simulink model "EGRVlv_DD"  (R2020b)
settings: configuration reference "cs_ert" (kept outside this file)
values from neighbouring files (symbols this model uses):
  EGRVlv_rPwmOutMax_C = 0.0    [EGRVlv_DD.sldd]
  EGRVlv_rPwmOutMin_C = 0.0    [EGRVlv_DD.sldd]
  EGRVlv_tiPs_C = 0.0    [EGRVlv_DD.sldd]
libraries: simulink x1
settings Model: DataDictionary=EGRVlv_DD.sldd  EnableAccessToBaseWorkspace=off  Creator=zhoutinglin  LastModifiedBy=zhoutinglin
settings ConfigSetRef: SourceName=cs_ert

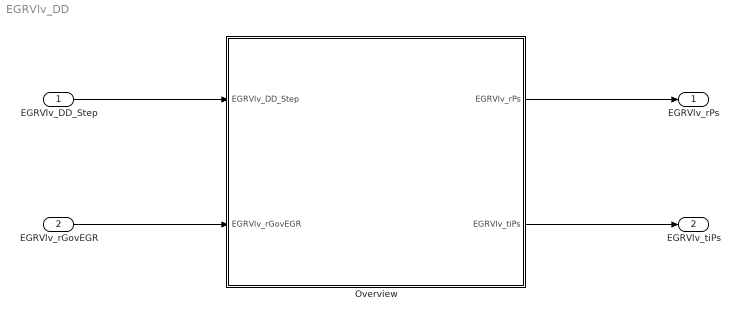
== system EGRVlv_DD ==
  EGRVlv_DD_Step : Inport  OutputFunctionCall=on
  EGRVlv_rGovEGR : Inport  Description=Control value for the EGR valve  Port=2  OutMin=-100  OutMax=100  OutDataTypeStr=DutyCycle  Unit=%  PortDimensions=[1 1]
  Overview : Subsystem
  EGRVlv_rPs : Outport  Description=Duty cycle to power stage  OutMin=-100  OutMax=100  OutDataTypeStr=DutyCycle  Unit=%  PortDimensions=[1 1]  VectorParamsAs1DForOutWhenUnconnected=off
  EGRVlv_tiPs : Outport  Description=signal period duration  Port=2  OutMin=0  OutMax=1000  OutDataTypeStr=Period_us1  Unit=us  PortDimensions=[1 1]  VectorParamsAs1DForOutWhenUnconnected=off
  wires:
  EGRVlv_DD_Step/1 -> Overview/1(EGRVlv_DD_Step)
  EGRVlv_rGovEGR/1 -> Overview/2(EGRVlv_rGovEGR)
  Overview/1(EGRVlv_rPs) -> EGRVlv_rPs/1
  Overview/2(EGRVlv_tiPs) -> EGRVlv_tiPs/1

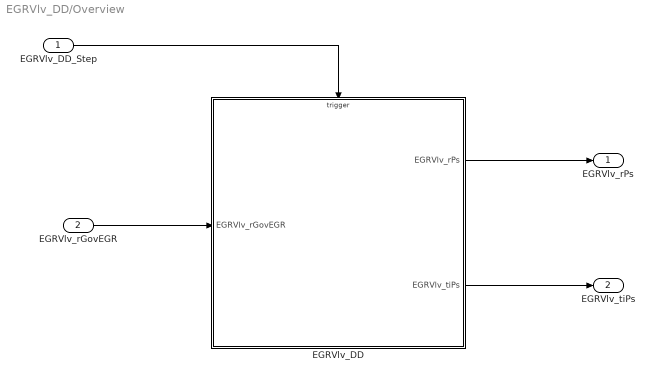
== system EGRVlv_DD/Overview ==
  EGRVlv_DD_Step : Inport
  EGRVlv_rGovEGR : Inport  Tag=%  Description=Control value for the EGR valve  Port=2  OutMin=-100  OutMax=100  OutDataTypeStr=DutyCycle  Unit=%  PortDimensions=[1 1]
  EGRVlv_DD : Subsystem
  EGRVlv_rPs : Outport  Tag=%  VectorParamsAs1DForOutWhenUnconnected=off
  EGRVlv_tiPs : Outport  Tag=us  Port=2  VectorParamsAs1DForOutWhenUnconnected=off
  wires:
  EGRVlv_DD/1(EGRVlv_rPs) -> EGRVlv_rPs/1
  EGRVlv_rGovEGR/1 -> EGRVlv_DD/1(EGRVlv_rGovEGR)
  EGRVlv_DD/2(EGRVlv_tiPs) -> EGRVlv_tiPs/1
  EGRVlv_DD_Step/1 -> EGRVlv_DD/Trigger

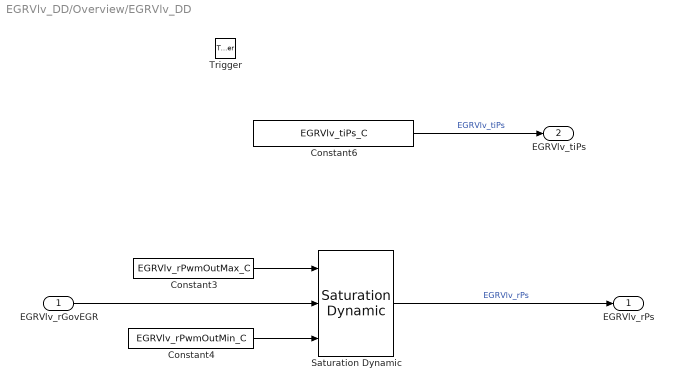
== system EGRVlv_DD/Overview/EGRVlv_DD ==
  EGRVlv_rGovEGR : Inport  Tag=%
  Trigger : TriggerPort  TriggerType=function-call  VariantControl=Variant  PortDimensions=1
  Constant3 : Constant  Value=EGRVlv_rPwmOutMax_C  SampleTime=-1
  Constant4 : Constant  Value=EGRVlv_rPwmOutMin_C  SampleTime=-1
  Constant6 : Constant  Value=EGRVlv_tiPs_C  SampleTime=-1
  Saturation Dynamic : simulink/Discontinuities/Saturation Dynamic  OutMin=[]  OutMax=[]  OutDataTypeStr=Inherit: Same as second input  OutDataType=fixdt(1, 16)  OutScaling=2^-10  DoSatur=off
  EGRVlv_rPs : Outport  Tag=kPa  VectorParamsAs1DForOutWhenUnconnected=off
  EGRVlv_tiPs : Outport  Tag=%  Port=2  VectorParamsAs1DForOutWhenUnconnected=off
  wires:
  Constant6/1 -> EGRVlv_tiPs/1  "EGRVlv_tiPs"
  Saturation Dynamic/1 -> EGRVlv_rPs/1  "EGRVlv_rPs"
  EGRVlv_rGovEGR/1 -> Saturation Dynamic/2
  Constant3/1 -> Saturation Dynamic/1
  Constant4/1 -> Saturation Dynamic/3
